simulink model "pendule_inv_etu"  (R2021a)
settings: Solver=VariableStepAuto  StartTime=0.0  StopTime=10.0  RelTol=1e-3
settings Model: Creator=hlafargu  LastModifiedBy=hlafargu

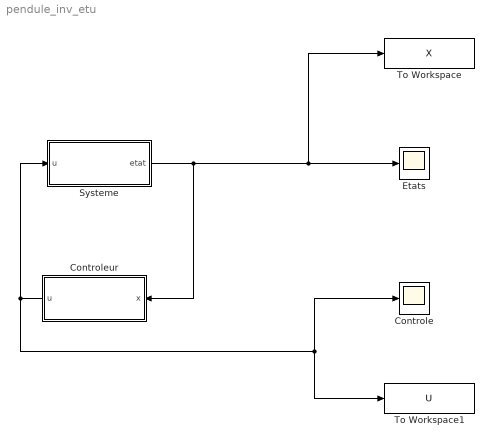
== system pendule_inv_etu ==
  Controle : Scope
  Controleur : Subsystem
  Etats : Scope
  Systeme : Subsystem
  To Workspace : ToWorkspace  VariableName=X  SaveFormat=Timeseries  SampleTime=-1
  To Workspace1 : ToWorkspace  VariableName=U  SaveFormat=Timeseries  SampleTime=-1
  wires:
  Systeme/1(etat) -> Controleur/1(x), To Workspace/1, Etats/1
  Controleur/1(u) -> To Workspace1/1, Controle/1, Systeme/1(u)

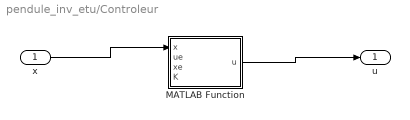
== system pendule_inv_etu/Controleur ==
  x : Inport
  MATLAB Function : MATLAB Function  TreatAsAtomicUnit=on
  u : Outport
  wires:
  x/1 -> MATLAB Function/1(x)
  MATLAB Function/1(u) -> u/1

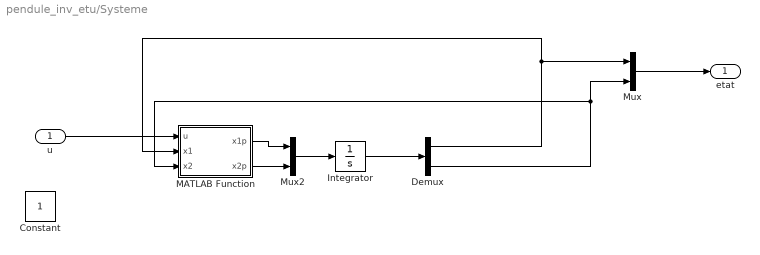
== system pendule_inv_etu/Systeme ==
  u : Inport
  Constant : Constant
  Demux : Demux  Outputs=2
  Integrator : Integrator
  MATLAB Function : MATLAB Function  TreatAsAtomicUnit=on
  Mux : Mux  Inputs=2
  Mux2 : Mux  Inputs=2
  etat : Outport
  wires:
  MATLAB Function/1(x1p) -> Mux2/1
  Mux/1 -> etat/1
  Demux/1 -> MATLAB Function/2(x1), Mux/1
  Integrator/1 -> Demux/1
  Demux/2 -> Mux/2, MATLAB Function/3(x2)
  MATLAB Function/2(x2p) -> Mux2/2
  Mux2/1 -> Integrator/1
  u/1 -> MATLAB Function/1(u)

== matlab function pendule_inv_etu/Systeme/MATLAB Function ==
  data: u input; x1p output; x1 input; x2 input; x2p output
function [x1p, x2p] = fcn(u,x1,x2)
x1p = x2;
x2p = g/l * sin(x1) - cos(x1) * u / l;

== matlab function pendule_inv_etu/Controleur/MATLAB Function ==
  data: x input; u output; ue input; xe input; K input
function u = fcn(x,ue, xe, K)

u = ue + K * (x-xe);
